simulink model "main_RI_LIEKF"  (R2023a)
settings: Solver=FixedStepAuto  StartTime=0.0  StopTime=220  FixedStep=0.01  RelTol=1e-3
InitFcn:
  | initNavigation0612_AOA;
values from neighbouring files (symbols this model uses):
  CF_enable = 0    [initNavigation.m]
  dt = 0.01    [initNavigation.m]
  dtDelay = -0.03    [initNavigation.m]
  g0 = 9.795    [initNavigation.m]
  gam0_rad = 0/57.3    (= 0)    [initNavigation.m]
  H_sensor_type = 0    [initNavigation.m]
  KF_enable = 1    [initNavigation.m]
  P0 = diag([1*ones(3,1);0.01*ones(3,1);0.1*ones(3,1);0.001*ones(3,1);0.00001*ones(3,1)])    [initNavigation.m]
  P0_RIEKF = diag([1*ones(3,1);0.01*ones(3,1);0.1*ones(3,1);0.001*ones(3,1);0.00001*ones(3,1);      0.01*ones(3,1);[0;2;2]/57.3;[0.1;0.1;0.1]])^2    [initNavigation.m]
  pd0 = 0    [initNavigation.m]
  pe0 = 0    [initNavigation.m]
  phi0_rad = 0/57.3    (= 0)    [initNavigation.m]
  pn0 = 0    [initNavigation.m]
  psi = -178    [initNavigation.m]
  psi0_rad = 0/57.3    (= 0)    [initNavigation.m]
  state_dim = 24    [initNavigation.m]
  Time = 0:0.01:(size(traindata.AttackAngle,1) - 1)*0.01    [NNLiftCoefficientFit.m]
  vd0 = 0    [initNavigation.m]
  ve0 = 0    [initNavigation.m]
  vn0 = 0    [initNavigation.m]
undefined symbols (not defined in the file or in its folder): DiscIntNeverNeededParam, Discrete, INS_CONST, INS_EXPORT, INS_PARAM, magnitude, p, param, pInitialization, sys
libraries: simulink x69, simulink_extras x64, dspstat3 x56, sharedtransform x49, ctrlSharedLib x36, sharedTrackingLibrary x17, FMT_Model_Lib x13, matrix_library x12, deeplib x4, dspsolvers x4, vrlib x4, aerolibconvert2 x1
(part 18 of 22)

== system main_RI_LIEKF/State estimation/distribute CF/distribute CF/Translation_estimate/V_Horizontal_estimation/Rxy_kalman filter1/Vxy kalman filter/kalman/Subsystem ==
  F : Inport
  G : Inport  Port=2
  Q : Inport  Port=3
  X : Inport  Port=4
  P : Inport  Port=5
  Add : Sum
  Math Function3 : Math  Operator=transpose  SignedPower=on
  Math Function4 : Math  Operator=transpose  SignedPower=on
  MatrixMultiply : Product  Multiplication=Matrix(*)
  MatrixMultiply1 : Product  Inputs=3  Multiplication=Matrix(*)
  MatrixMultiply8 : Product  Inputs=3  Multiplication=Matrix(*)
  Xk_k_1 : Outport
  Pk_k_1 : Outport  Port=2
  wires:
  [Pk_k_1] -> Pk_k_1/1
  [Xk_k_1] -> Xk_k_1/1
  P/1 -> [P]
  X/1 -> [X]
  Q/1 -> [Q]
  G/1 -> [G]
  F/1 -> [F]
  [F] -> MatrixMultiply/1
  [G] -> Math Function4/1
  [X] -> MatrixMultiply/2
  MatrixMultiply8/1 -> Add/2
  [G] -> MatrixMultiply8/1
  Add/1 -> [Pk_k_1]
  [F] -> MatrixMultiply1/1
  [P] -> MatrixMultiply1/2
  Math Function3/1 -> MatrixMultiply1/3
  [F] -> Math Function3/1
  MatrixMultiply1/1 -> Add/1
  MatrixMultiply/1 -> [Xk_k_1]
  [Q] -> MatrixMultiply8/2
  Math Function4/1 -> MatrixMultiply8/3

== system main_RI_LIEKF/State estimation/distribute CF/distribute CF/Translation_estimate/V_Horizontal_estimation/Rxy_kalman filter1/Vxy kalman filter/kalman/Subsystem1 ==
  note: 计算卡尔曼增益Kk
  Xkk : Inport
  Pkk : Inport  Port=2
  H : Inport  Port=3
  R : Inport  Port=4
  Z : Inport  Port=5
  Enable : EnablePort
  Add2 : Sum
  Add3 : Sum  Inputs=+-
  Add4 : Sum  Inputs=+-
  Add5 : Sum
  Constant : Constant  Value=eye(4)  OutDataTypeStr=single
  LDL Solver1 : dspsolvers/LDL Solver  errmode=Warning
      settings: RTWMemSecFuncInitTerm=Default  RTWMemSecFuncExecute=Default  RTWMemSecDataConstants=Default  RTWMemSecDataInternal=Default  RTWMemSecDataParameters=Default
  Math Function5 : Math  Operator=transpose  SignedPower=on
  Math Function6 : Math  Operator=transpose  SignedPower=on
  MatrixMultiply{4..7,9..10} (6 alike) : Product  Multiplication=Matrix(*)
  Scope : Scope
  POut : Outport
  XOut : Outport  Port=2
  wires:
  Pkk/1 -> [Pk_k_1]
  Z/1 -> [Z]
  Xkk/1 -> [Xk_k_1]
  Add2/1 -> XOut/1
  H/1 -> [H]
  MatrixMultiply6/1 -> Add4/2
  Add5/1 -> LDL Solver1/1
  R/1 -> [R]
  [Pk_k_1] -> MatrixMultiply7/2
  [Xk_k_1] -> MatrixMultiply9/2
  [H] -> MatrixMultiply9/1
  [H] -> MatrixMultiply6/2
  [Xk_k_1] -> Add2/1
  [Kk] -> MatrixMultiply6/1
  Constant/1 -> Add4/1
  [R] -> Add5/2
  [Pk_k_1] -> MatrixMultiply10/2
  [H] -> Math Function5/1
  LDL Solver1/1 -> Math Function6/1
  MatrixMultiply5/1 -> Add5/1
  MatrixMultiply10/1 -> LDL Solver1/2, MatrixMultiply5/1
  [Z] -> Add3/1
  [Kk] -> MatrixMultiply4/1
  MatrixMultiply4/1 -> Add2/2
  Add4/1 -> MatrixMultiply7/1
  Math Function6/1 -> [Kk], Scope/1
  Math Function5/1 -> MatrixMultiply5/2
  Add3/1 -> MatrixMultiply4/2
  [H] -> MatrixMultiply10/1
  MatrixMultiply7/1 -> POut/1
  MatrixMultiply9/1 -> Add3/2

== system main_RI_LIEKF/State estimation/distribute CF/distribute CF/AHRS1/Correct/Attitude_Correction/Attitude_Correct/Acc_Correct/Verticle_Correct/Saturation ==
  u : Inport
  Constant1 : Constant  Value=1e-4  OutDataTypeStr=Inherit: Inherit via back propagation
  Divide : Product  Inputs=**/
  Divide1 : Product  Inputs=*/
  Divide2 : Product  Inputs=**
  MinMax : MinMax  Function=max  Inputs=2
  Saturation : Saturate  UpperLimit=pi/2  LowerLimit=-pi/2
  Trigonometric Function : Trigonometry
  Vector Modulus : FMT_Model_Lib/Math/Vector Modulus
  max : Constant  Value=10/180*pi  OutDataTypeStr=single
  y : Outport
  wires:
  Constant1/1 -> MinMax/2
  Saturation/1 -> Trigonometric Function/1
  u/1 -> Vector Modulus/1, Divide/1
  Trigonometric Function/1 -> Divide2/1
  Divide/1 -> y/1
  Vector Modulus/1 -> Divide1/1, MinMax/1
  Divide1/1 -> Saturation/1
  Divide2/1 -> Divide/2
  max/1 -> Divide1/2, Divide2/2
  MinMax/1 -> Divide/3

== system main_RI_LIEKF/State estimation/distribute CF/distribute CF/AHRS1/Correct/Attitude_Correction/Attitude_Correct/Acc_Estimator/Measure_Acc/Bus_Selection ==
  Sensor_Data : Inport
  Bus Selector2 : BusSelector  OutputSignals=GPS_Data.vn_mPs,GPS_Data.ve_mPs,GPS_Data.vd_mPs
  Mux : Mux  Inputs=3
  gps_vel_O_mPs : Outport
  wires:
  Sensor_Data/1 -> Bus Selector2/1
  Bus Selector2/1 -> Mux/1  "<vn_mPs>"
  Bus Selector2/2 -> Mux/2  "<ve_mPs>"
  Bus Selector2/3 -> Mux/3  "<vd_mPs>"
  Mux/1 -> gps_vel_O_mPs/1

== system main_RI_LIEKF/State estimation/distribute CF/distribute CF/AHRS1/Correct/Attitude_Correction/Attitude_Correct/Acc_Estimator/Measure_Acc/GPS_Meas_Acc ==
  reset : Inport
  gps_vel_O_mPs : Inport  Port=2
  Enable : EnablePort  StatesWhenEnabling=reset
  Integrator : DiscreteIntegrator  ExternalReset=level  SampleTime=-1  ICPrevOutput=DiscIntNeverNeededParam  ICPrevScaledInput=DiscIntNeverNeededParam
  Integrator1 : DiscreteIntegrator  ExternalReset=level  InitialConditionSource=external  SampleTime=-1  ICPrevOutput=DiscIntNeverNeededParam  ICPrevScaledInput=DiscIntNeverNeededParam
  Sum : Sum  Inputs=|++
  Sum1 : Sum  Inputs=|+-
  gain : Gain  Gain=2*zeta*fc
  gain1 : Gain  Gain=fc^2
  gps_acc_O_mPs2 : Outport
  wires:
  Integrator1/1 -> Sum1/2
  Integrator/1 -> gps_acc_O_mPs2/1, Sum/2
  reset/1 -> Integrator1/2, Integrator/2
  gain/1 -> Sum/1
  Sum1/1 -> gain/1, gain1/1
  Sum/1 -> Integrator1/1
  gps_vel_O_mPs/1 -> Sum1/1, Integrator1/3
  gain1/1 -> Integrator/1

== system main_RI_LIEKF/State estimation/distribute CF/distribute CF/AHRS1/Correct/Attitude_Correction/Attitude_Correct/Acc_Estimator/Measure_Acc/Valid_Check ==
  Sensor_Data : Inport
  Bus Selector : BusSelector  OutputSignals=GPS_Data.GPS_valid,GPS_Data.spd_quality
  Logical Operator1 : Logic  AllPortsSameDT=off  OutDataTypeStr=boolean
  Relay : Relay  OnSwitchValue=0.2  OffSwitchValue=0.1
  gps_meas_acc_valid : Outport
  wires:
  Sensor_Data/1 -> Bus Selector/1
  Logical Operator1/1 -> gps_meas_acc_valid/1
  Bus Selector/1 -> Logical Operator1/1  "<GPS_valid>"
  Relay/1 -> Logical Operator1/2
  Bus Selector/2 -> Relay/1  "<spd_quality>"

== system main_RI_LIEKF/State estimation/distribute CF/distribute CF/Correct/Attitude_Correction/Attitude_Correct/Acc_Correct/Verticle_Correct/Saturation/norm ==
  In1 : Inport
  Sqrt : Sqrt
  Square : Math  Operator=square  SignedPower=on
  Sum of Elements : Sum  Inputs=+
  Out1 : Outport
  wires:
  Sum of Elements/1 -> Sqrt/1
  Square/1 -> Sum of Elements/1
  Sqrt/1 -> Out1/1
  In1/1 -> Square/1

== system main_RI_LIEKF/State estimation/distribute CF/distribute CF/Correct/Attitude_Correction/Attitude_Correct/Subsystem2/gps_meas_acc-加速度估计/TD_baro/Subsystem ==
  In1 : Inport
  Constant1 : Constant  Value=dt  OutDataTypeStr=single
  Constant3 : Constant  Value=0.23  OutDataTypeStr=single
  Constant4 : Constant  Value=900  OutDataTypeStr=single
  Delay1 : Delay  DelayLength=1  InitialConditionSource=Input port
      settings: InputPortMap=u0,p4
  MATLAB Function2 : MATLAB Function  TreatAsAtomicUnit=on
  Memory : Memory  InheritSampleTime=on
  Scope : Scope  NumInputPorts=3
  u2 : Outport
  wires:
  In1/1 -> MATLAB Function2/2(u0), Delay1/2, Scope/1
  Constant1/1 -> MATLAB Function2/1(T)
  MATLAB Function2/1(u1) -> Delay1/1
  Memory/1 -> Scope/2, MATLAB Function2/4("u2 ")
  Constant3/1 -> MATLAB Function2/5(h)
  Delay1/1 -> MATLAB Function2/3("u1 "), Scope/3
  MATLAB Function2/2(u2) -> u2/1, Memory/1
  Constant4/1 -> MATLAB Function2/6(r)

== system main_RI_LIEKF/State estimation/distribute CF/distribute CF/Correct/Attitude_Correction/Attitude_Correct/Subsystem2/gps_meas_acc-加速度估计/TD_baro/Subsystem1 ==
  In1 : Inport
  Constant1 : Constant  Value=dt  OutDataTypeStr=single
  Constant3 : Constant  Value=0.23  OutDataTypeStr=single
  Constant4 : Constant  Value=900  OutDataTypeStr=single
  Delay1 : Delay  DelayLength=1  InitialConditionSource=Input port
      settings: InputPortMap=u0,p4
  MATLAB Function2 : MATLAB Function  TreatAsAtomicUnit=on
  Memory : Memory  InheritSampleTime=on
  Scope : Scope  NumInputPorts=3
  u2 : Outport
  wires:
  Constant4/1 -> MATLAB Function2/6(r)
  MATLAB Function2/2(u2) -> u2/1, Memory/1
  Delay1/1 -> Scope/3, MATLAB Function2/3("u1 ")
  Constant3/1 -> MATLAB Function2/5(h)
  Memory/1 -> MATLAB Function2/4("u2 "), Scope/2
  MATLAB Function2/1(u1) -> Delay1/1
  Constant1/1 -> MATLAB Function2/1(T)
  In1/1 -> Scope/1, Delay1/2, MATLAB Function2/2(u0)

== system main_RI_LIEKF/State estimation/distribute CF/distribute CF/Correct/Attitude_Correction/Attitude_Correct/Subsystem2/gps_meas_acc-加速度估计/TD_baro/Subsystem2 ==
  In1 : Inport
  Constant1 : Constant  Value=dt  OutDataTypeStr=single
  Constant3 : Constant  Value=0.23  OutDataTypeStr=single
  Constant4 : Constant  Value=900  OutDataTypeStr=single
  Delay1 : Delay  DelayLength=1  InitialConditionSource=Input port
      settings: InputPortMap=u0,p4
  MATLAB Function2 : MATLAB Function  TreatAsAtomicUnit=on
  Memory : Memory  InheritSampleTime=on
  Scope : Scope  NumInputPorts=3
  u2 : Outport
  wires:
  In1/1 -> MATLAB Function2/2(u0), Delay1/2, Scope/1
  Constant1/1 -> MATLAB Function2/1(T)
  MATLAB Function2/1(u1) -> Delay1/1
  Memory/1 -> Scope/2, MATLAB Function2/4("u2 ")
  Constant3/1 -> MATLAB Function2/5(h)
  Delay1/1 -> MATLAB Function2/3("u1 "), Scope/3
  MATLAB Function2/2(u2) -> u2/1, Memory/1
  Constant4/1 -> MATLAB Function2/6(r)

== matlab function main_RI_LIEKF/State estimation/15dim KF1/Error State Kalman Filter/MATLAB Function2 ==
  data: P output
function P=P0
    g0 = 9.7803267714;       % 重力加速度
    %t=0.01;                  %采样时间
    sec = 4.848136811095360e-06;
    Re = 6378137;
    dph = 4.848136811095360e-06;
    ug = 9.780326771399999e-06;

    %角度随机游走系数(度/小时)
    % web=[3;3;3]*(pi/180)/3600;
     %web=[6;6;6]*sec;
     web= [2.908882086657216e-07;2.908882086657216e-07;2.908882086657216e-07];
    %速度随机游走系数（米/s/sqrt（小时））
     %wdb=[500;500;500]*ug;
    wdb=[9.780326771400000e-06;9.780326771400000e-06;9.780326771400000e-06];

    %sqg=[1;1;1]*(pi/180)/3600;
    %sqa=[1;1;1]*1e-6*g0;
    
    sqg=zeros(3,1);
    sqa=zeros(3,1);
    %系统噪声协方差矩阵
    %kf.Qt = diag([imuerr.web; imuerr.wdb; zeros(3,1); imuerr.sqg; imuerr.sqa; zeros(3,1)])^2;
 %Q=diag([web;wdb;zeros(3,1);sqg;sqa;w_GPS_V;w_GPS_R])^2;
%  Q=diag([web;wdb;zeros(3,1);sqg;sqa])^2;
  P = diag([1*ones(3,1);0.1*ones(3,1);[0.001;0.001;0.01];0.001*ones(3,1);0.1*ones(3,1)]);
%P = 1e-3^2*ones(15,1);
%Q = diag([8.461594994075240e-10*[1;1;1];9.565479175536352e-09*[1;1;1];zeros(15,1)]);
end

== matlab function main_RI_LIEKF/State estimation/15dim KF1/INS propogation/Init_PVQ2/Horizontal_attitude/Hem2JPL ==
  data: q input; y output
function y = fcn(q)

y = [q(2:4);q(1)];

== matlab function main_RI_LIEKF/State estimation/15dim KF1/INS propogation/Init_PVQ2/Horizontal_attitude/Hem2JPL1 ==
  data: q input; y output
function y = fcn(q)

y = [q(2:4);q(1)];

== matlab function main_RI_LIEKF/State estimation/15dim KF1/INS propogation/att_update/JPLQuatMult ==
  data: quatA input; q_t output; quatB input
function q_t = QuatMult(quatA,quatB)
% Calculate the following quaternion product quatA * quatB using the 
% standard identity 
%{
inline Eigen::Matrix<double, 4, 1> quat_multiply(const Eigen::Matrix<double, 4, 1> &q, const Eigen::Matrix<double, 4, 1> &p) {
  Eigen::Matrix<double, 4, 1> q_t;
  Eigen::Matrix<double, 4, 4> Qm;
  // create big L matrix
  Qm.block(0, 0, 3, 3) = q(3, 0) * Eigen::MatrixXd::Identity(3, 3) - skew_x(q.block(0, 0, 3, 1));
  Qm.block(0, 3, 3, 1) = q.block(0, 0, 3, 1);
  Qm.block(3, 0, 1, 3) = -q.block(0, 0, 3, 1).transpose();
  Qm(3, 3) = q(3, 0);
  q_t = Qm * p;
  // ensure unique by forcing q_4 to be >0
  if (q_t(3, 0) < 0) {
    q_t *= -1;
  }
  // normalize and return
  return q_t / q_t.norm();
}
%}
Qm = zeros(4,4);
q_t = zeros(4,1);
Qm(1:3,1:3) = quatA(4)*eye(3,3) - skewMat(quatA(1:3));
Qm(1:3,4) = quatA(1:3);
Qm(4,1:3) = -quatA(1:3)';
Qm(4,4) = quatA(4);
q_t = Qm * quatB;
if q_t(4) < 0
    q_t = q_t * (-1);
end
q_t = q_t / norm(q_t);
end

== matlab function main_RI_LIEKF/State estimation/15dim KF1/INS propogation/att_update/JPLQuatMult1 ==
  data: quatA input; q_t output; quatB input
function q_t = QuatMult(quatA,quatB)
% Calculate the following quaternion product quatA * quatB using the 
% standard identity 
%{
inline Eigen::Matrix<double, 4, 1> quat_multiply(const Eigen::Matrix<double, 4, 1> &q, const Eigen::Matrix<double, 4, 1> &p) {
  Eigen::Matrix<double, 4, 1> q_t;
  Eigen::Matrix<double, 4, 4> Qm;
  // create big L matrix
  Qm.block(0, 0, 3, 3) = q(3, 0) * Eigen::MatrixXd::Identity(3, 3) - skew_x(q.block(0, 0, 3, 1));
  Qm.block(0, 3, 3, 1) = q.block(0, 0, 3, 1);
  Qm.block(3, 0, 1, 3) = -q.block(0, 0, 3, 1).transpose();
  Qm(3, 3) = q(3, 0);
  q_t = Qm * p;
  // ensure unique by forcing q_4 to be >0
  if (q_t(3, 0) < 0) {
    q_t *= -1;
  }
  // normalize and return
  return q_t / q_t.norm();
}
%}
Qm = zeros(4,4);
q_t = zeros(4,1);
Qm(1:3,1:3) = quatA(4)*eye(3,3) - skewMat(quatA(1:3));
Qm(1:3,4) = quatA(1:3);
Qm(4,1:3) = -quatA(1:3)';
Qm(4,4) = quatA(4);
q_t = Qm * quatB;
if q_t(4) < 0
    q_t = q_t * (-1);
end
q_t = q_t / norm(q_t);
end

== matlab function main_RI_LIEKF/State estimation/15dim KF1/INS propogation/att_update/JPLrv2q ==
  data: rotVec input; quaternion output
% convert froma rotation vector in radians to a quaternion
function quaternion = RotToQuat(rotVec)

vecLength = sqrt(rotVec(1)^2 + rotVec(2)^2 + rotVec(3)^2);

if vecLength < 1e-6
  quaternion = [0;0;0;1];
else
  quaternion = [rotVec/vecLength*sin(0.5*vecLength);cos(0.5*vecLength);];
end

== matlab function main_RI_LIEKF/State estimation/15dim KF1/INS propogation/att_update/JPLrv2q1 ==
  data: deltaTheta input; updateQuat output
% convert froma rotation vector in radians to a quaternion
function updateQuat = RotToQuat(deltaTheta)

    deltaq = 0.5 * deltaTheta;
    
    checkNorm = deltaq' * deltaq;
    
    if checkNorm > 1
        updateQuat = [deltaq; 1];
        updateQuat = updateQuat / sqrt(1 + checkNorm);
    else
        updateQuat = [deltaq; sqrt(1 - checkNorm)];
    end
    
    updateQuat = updateQuat / norm(updateQuat);
end

== matlab function main_RI_LIEKF/State estimation/15dim KF1/INS propogation/att_update/MATLAB Function1 ==
  data: q input; Rot output
function Rot = quat_2_Rot(q)

%{
inline Eigen::Matrix<double, 3, 3> quat_2_Rot(const Eigen::Matrix<double, 4, 1> &q) {
  Eigen::Matrix<double, 3, 3> q_x = skew_x(q.block(0, 0, 3, 1));
  Eigen::MatrixXd Rot = (2 * std::pow(q(3, 0), 2) - 1) * Eigen::MatrixXd::Identity(3, 3) - 2 * q(3, 0) * q_x +
                        2 * q.block(0, 0, 3, 1) * (q.block(0, 0, 3, 1).transpose());
  return Rot;
}
%}
q_x = skewMat(q(1:3));
Rot = (2 * q(4)^2 - 1) * eye(3, 3) - 2 * q(4) * q_x +...
       2 * q(1:3) * q(1:3)';
end

== matlab function main_RI_LIEKF/State estimation/RI EKF/INS propogation/AOA//SA//Vwind update/Subsystem/LSTM predict1/MATLAB Function5 ==
  data: X input; X_nYPred output
function X_nYPred = LSTMnet(X)
    sig_X = [0.2380; 0.1523 ;0.0429;0.1379];
    sig_Y = 0.0690;
    mu_X = [0.0068;-0.0055;-0.0070;-0.0450];
    mu_Y = -0.0228;
    X_norm = (X - mu_X) ./ sig_X;
    persistent X_nYPredorm_store;
    if isempty(X_nYPredorm_store)
        X_nYPredorm_store = zeros(1000,4);
    end

    X_nYPredorm_store = [X_nYPredorm_store(2:end,:);X_norm'];
    %[~,YPred_seq] = predictAndUpdateState(net.net,X_nYPredorm_store);
     X_nYPred = single(X_nYPredorm_store);
    % YPred_seq = predict(net.net,X_nYPredorm_store');
    % YPred_test = YPred_seq(end);
    % YPred_test = double(YPred_test* sig_Y + mu_Y)*57.3;

end

== matlab function main_RI_LIEKF/State estimation/ER EKF/INS propogation/Init_PVQ/Horizontal_attitude/Hem2JPL ==
  data: q input; y output
function y = fcn(q)

y = [q(2:4);q(1)];

== matlab function main_RI_LIEKF/State estimation/ER EKF/INS propogation/Init_PVQ/Horizontal_attitude/Hem2JPL1 ==
  data: q input; y output
function y = fcn(q)

y = [q(2:4);q(1)];

== matlab function main_RI_LIEKF/State estimation/0609bk/Error State Kalman Filter/Extended Kalman Filter1/Output/MATLAB Function ==
  data: S input; P output
function P = fcn(S)
    
    % Get back Covariance from Square-root Covariance
    P = S*S';
    
end

== matlab function main_RI_LIEKF/State estimation/ER EKF/INS propogation/att_update/JPLQuatMult ==
  data: quatA input; q_t output; quatB input
function q_t = QuatMult(quatA,quatB)
% Calculate the following quaternion product quatA * quatB using the 
% standard identity 
%{
inline Eigen::Matrix<double, 4, 1> quat_multiply(const Eigen::Matrix<double, 4, 1> &q, const Eigen::Matrix<double, 4, 1> &p) {
  Eigen::Matrix<double, 4, 1> q_t;
  Eigen::Matrix<double, 4, 4> Qm;
  // create big L matrix
  Qm.block(0, 0, 3, 3) = q(3, 0) * Eigen::MatrixXd::Identity(3, 3) - skew_x(q.block(0, 0, 3, 1));
  Qm.block(0, 3, 3, 1) = q.block(0, 0, 3, 1);
  Qm.block(3, 0, 1, 3) = -q.block(0, 0, 3, 1).transpose();
  Qm(3, 3) = q(3, 0);
  q_t = Qm * p;
  // ensure unique by forcing q_4 to be >0
  if (q_t(3, 0) < 0) {
    q_t *= -1;
  }
  // normalize and return
  return q_t / q_t.norm();
}
%}
Qm = zeros(4,4);
q_t = zeros(4,1);
Qm(1:3,1:3) = quatA(4)*eye(3,3) - skewMat(quatA(1:3));
Qm(1:3,4) = quatA(1:3);
Qm(4,1:3) = -quatA(1:3)';
Qm(4,4) = quatA(4);
q_t = Qm * quatB;
if q_t(4) < 0
    q_t = q_t * (-1);
end
q_t = q_t / norm(q_t);
end

== matlab function main_RI_LIEKF/State estimation/ER EKF/INS propogation/att_update/JPLQuatMult1 ==
  data: quatA input; q_t output; quatB input
function q_t = QuatMult(quatA,quatB)
% Calculate the following quaternion product quatA * quatB using the 
% standard identity 
%{
inline Eigen::Matrix<double, 4, 1> quat_multiply(const Eigen::Matrix<double, 4, 1> &q, const Eigen::Matrix<double, 4, 1> &p) {
  Eigen::Matrix<double, 4, 1> q_t;
  Eigen::Matrix<double, 4, 4> Qm;
  // create big L matrix
  Qm.block(0, 0, 3, 3) = q(3, 0) * Eigen::MatrixXd::Identity(3, 3) - skew_x(q.block(0, 0, 3, 1));
  Qm.block(0, 3, 3, 1) = q.block(0, 0, 3, 1);
  Qm.block(3, 0, 1, 3) = -q.block(0, 0, 3, 1).transpose();
  Qm(3, 3) = q(3, 0);
  q_t = Qm * p;
  // ensure unique by forcing q_4 to be >0
  if (q_t(3, 0) < 0) {
    q_t *= -1;
  }
  // normalize and return
  return q_t / q_t.norm();
}
%}
Qm = zeros(4,4);
q_t = zeros(4,1);
Qm(1:3,1:3) = quatA(4)*eye(3,3) - skewMat(quatA(1:3));
Qm(1:3,4) = quatA(1:3);
Qm(4,1:3) = -quatA(1:3)';
Qm(4,4) = quatA(4);
q_t = Qm * quatB;
if q_t(4) < 0
    q_t = q_t * (-1);
end
q_t = q_t / norm(q_t);
end

== matlab function main_RI_LIEKF/State estimation/ER EKF/INS propogation/att_update/JPLrv2q ==
  data: rotVec input; quaternion output
% convert froma rotation vector in radians to a quaternion
function quaternion = RotToQuat(rotVec)

vecLength = sqrt(rotVec(1)^2 + rotVec(2)^2 + rotVec(3)^2);

if vecLength < 1e-6
  quaternion = [0;0;0;1];
else
  quaternion = [rotVec/vecLength*sin(0.5*vecLength);cos(0.5*vecLength);];
end

== matlab function main_RI_LIEKF/State estimation/ER EKF/INS propogation/att_update/JPLrv2q1 ==
  data: deltaTheta input; updateQuat output
% convert froma rotation vector in radians to a quaternion
function updateQuat = RotToQuat(deltaTheta)

    deltaq = 0.5 * deltaTheta;
    
    checkNorm = deltaq' * deltaq;
    
    if checkNorm > 1
        updateQuat = [deltaq; 1];
        updateQuat = updateQuat / sqrt(1 + checkNorm);
    else
        updateQuat = [deltaq; sqrt(1 - checkNorm)];
    end
    
    updateQuat = updateQuat / norm(updateQuat);
end

== matlab function main_RI_LIEKF/State estimation/ER EKF/INS propogation/att_update/MATLAB Function1 ==
  data: q input; Rot output
function Rot = quat_2_Rot(q)

%{
inline Eigen::Matrix<double, 3, 3> quat_2_Rot(const Eigen::Matrix<double, 4, 1> &q) {
  Eigen::Matrix<double, 3, 3> q_x = skew_x(q.block(0, 0, 3, 1));
  Eigen::MatrixXd Rot = (2 * std::pow(q(3, 0), 2) - 1) * Eigen::MatrixXd::Identity(3, 3) - 2 * q(3, 0) * q_x +
                        2 * q.block(0, 0, 3, 1) * (q.block(0, 0, 3, 1).transpose());
  return Rot;
}
%}
q_x = skewMat(q(1:3));
Rot = (2 * q(4)^2 - 1) * eye(3, 3) - 2 * q(4) * q_x +...
       2 * q(1:3) * q(1:3)';
end

== matlab function main_RI_LIEKF/State estimation/bak1/Error State Kalman Filter/Simulink Function - State Transition Jacobian/Cal Phi/MATLAB Function1 ==
  data: axyz input; Phi output; Cnb input; wxyz input; dt input
function Phi = fcn(axyz, Cnb, wxyz,dt)
    
    %{
    F.block(0, 0, 3, 3) = exp_so3(-w_hat * dt);
        F.block(0, 9, 3, 3).noalias() = -exp_so3(-w_hat * dt) * Jr_so3(-w_hat * dt) * dt;
        F.block(9, 9, 3, 3).setIdentity();
        F.block(6, 0, 3, 3).noalias() = -R_Gtoi.transpose() * skew_x(a_hat * dt);
        F.block(6, 6, 3, 3).setIdentity();
        F.block(6, 12, 3, 3) = -R_Gtoi.transpose() * dt;
        F.block(12, 12, 3, 3).setIdentity();
        F.block(3, 0, 3, 3).noalias() = -0.5 * R_Gtoi.transpose() * skew_x(a_hat * dt * dt);
        F.block(3, 6, 3, 3) = Eigen::Matrix3d::Identity() * dt;
        F.block(3, 12, 3, 3) = -0.5 * R_Gtoi.transpose() * dt * dt;
        F.block(3, 3, 3, 3).setIdentity();
        Eigen::Matrix<double, 15, 12> G = Eigen::Matrix<double, 15, 12>::Zero();
    %}
    Phi = zeros(18,18);
    % 
    Phi(1:3,1:3) = eye(3);      %P-P
    Phi(1:3,4:6) = dt * eye(3); %P-V
    Phi(1:3,7:9) = -0.5*Cnb'*skewMat(axyz * dt * dt); %P-the
    % 
    Phi(4:6,4:6) = eye(3);
    Phi(4:6,7:9) = -Cnb' * skewMat(axyz * dt);
    Phi(4:6,10:12) = -Cnb'*dt ;
    % 
    Phi(7:9,7:9) = exp_so3(-wxyz * dt);     %the-the
    Phi(7:9,13:15) = -exp_so3(-wxyz * dt) * Jl_so3(wxyz * dt) * dt; %the-bias g
    % 
    Phi(10:12,10:12) = eye(3);
    % % 
    Phi(13:15,13:15) = eye(3);
    % 
    Phi(1:3,10:12) = - 0.5*Cnb' * dt * dt;
    Phi(16:18,16:18) = eye(3);
end

== matlab function main_RI_LIEKF/State estimation/bak1/Error State Kalman Filter/Simulink Function - State Transition Jacobian/MATLAB Function ==
  data: Cnb input; G output; wxyz input; dt input
function G = fcn(Cnb, wxyz, dt)
    % G.block(0, 0, 3, 3) = -exp_so3(-w_hat * dt) * Jr_so3(-w_hat * dt) * dt;
    %    G.block(6, 3, 3, 3) = -R_Gtoi.transpose() * dt;
    %    G.block(3, 3, 3, 3) = -0.5 * R_Gtoi.transpose() * dt * dt;
    %    G.block(9, 6, 3, 3).setIdentity();
    %    G.block(12, 9, 3, 3).setIdentity();
    
    G = zeros(18,15);
    G(7:9,4:6) = -exp_so3(-wxyz * dt) * Jl_so3(wxyz * dt) * dt;
    G(1:3,1:3) = -0.5 * Cnb' * dt * dt;
    G(4:6,1:3) = -Cnb' * dt;
    G(10:12,7:9) = eye(3);
    G(13:15,10:12) = eye(3);
    G(13:15,10:12) = eye(3);
    G(16:18,13:15) = eye(3);
    G(16:18,1:3) = -eye(3);
end

== matlab function main_RI_LIEKF/State estimation/bak1/INS propogation/att_update/MATLAB Function ==
  data: Rbn_k_1 input; Rbn output; w input; dt input
function Rbn = fcn(Rbn_k_1, w, dt)
    Rbn = Rbn_k_1 * exp_so3(w * dt);
end

== matlab function main_RI_LIEKF/State estimation/bak1/INS propogation/att_update/MATLAB Function2 ==
  data: delta input; Rbn_correct output single size=[3,3]; Rbn input
function Rbn_correct = fcn(delta, Rbn)
    Rbn_correct = zeros(3,3);
    Rbn_correct = exp_so3(delta)* Rbn;
end

== matlab function main_RI_LIEKF/Sensor_Data_Process/IMU_Data_Process/accl_preprocessing2/MATLAB Function1 ==
  data: curr_input input; curr_output output single; sample_freq input; cutoff_freq input
function curr_output = second_LPF_Butter_x(curr_input,sample_freq,cutoff_freq)
   persistent input_x;
   persistent output_x;

   if isempty(input_x)
       input_x = [0;0;0];
   end
   
   if isempty(output_x)
       output_x = [0;0;0];
   end
    B = [0,0,0];
    A = [0,0,0];
    M_PI_F = 3.1415926;
	fr = sample_freq / cutoff_freq;
	ohm = tan( M_PI_F / fr );
	c = 1.0 + 2.0 * cos( M_PI_F / 4.0 ) * ohm + ohm * ohm;
	B(1) = ohm * ohm / c;
	B(2) = 2.0 * B(1);
	B(3) = B(1);
	A(1) = 2.0 * ( ohm * ohm - 1.0) / c;
	A(2) = (1.0 - 2.0 * cos( M_PI_F / 4.0 ) * ohm + ohm * ohm) / c;
	%/*获取最新输入*/
	input_x(3) = curr_input;
	%/* Butterworth */
	output_x(3) =B(1) * input_x(3) + B(2) * input_x(2) +B(3) * input_x(1) - A(1) * output_x(2) - A(2) * output_x(1);
	curr_output = single(output_x(3));
   % /* 输入序列保存 */
	input_x(1) = input_x(2);
	input_x(2) = input_x(3);
	%/*输出序列保存 */
	output_x(1) = output_x(2);
	output_x(2) = output_x(3);

== matlab function main_RI_LIEKF/State estimation/bak1/INS propogation/vel_pos_update/pos update/MATLAB Function ==
  data: dtheta input; pos_correct output single; KFState_dp input; pos input
function pos_correct = fcn(dtheta, KFState_dp, pos)
    
    pos_correct =  KFState_dp + exp_so3(dtheta)*pos;
end

== matlab function main_RI_LIEKF/State estimation/bak1/INS propogation/vel_pos_update/vel update/MATLAB Function ==
  data: dtheta input; vel_correct output single; KFState_dv input; vel input
function vel_correct = fcn(dtheta, KFState_dv, vel)
    
    vel_correct =  KFState_dv + exp_so3( dtheta)*vel;
end

== matlab function main_RI_LIEKF/State estimation/RI EKF/Error State Kalman Filter/bak/Simulink Function - State Transition Jacobian/Cal Phi1/MATLAB Function1 ==
  data: vn input; Phi output; pn input; Rbn input; dt input
function Phi = fcn(vn,pn, Rbn,dt)
    
    %{
    F.block(0, 0, 3, 3) = exp_so3(-w_hat * dt);
        F.block(0, 9, 3, 3).noalias() = -exp_so3(-w_hat * dt) * Jr_so3(-w_hat * dt) * dt;
        F.block(9, 9, 3, 3).setIdentity();
        F.block(6, 0, 3, 3).noalias() = -R_Gtoi.transpose() * skew_x(a_hat * dt);
        F.block(6, 6, 3, 3).setIdentity();
        F.block(6, 12, 3, 3) = -R_Gtoi.transpose() * dt;
        F.block(12, 12, 3, 3).setIdentity();
        F.block(3, 0, 3, 3).noalias() = -0.5 * R_Gtoi.transpose() * skew_x(a_hat * dt * dt);
        F.block(3, 6, 3, 3) = Eigen::Matrix3d::Identity() * dt;
        F.block(3, 12, 3, 3) = -0.5 * R_Gtoi.transpose() * dt * dt;
        F.block(3, 3, 3, 3).setIdentity();
        Eigen::Matrix<double, 15, 12> G = Eigen::Matrix<double, 15, 12>::Zero();
    %}
    %
    %
    %F = [0_33         0_33  0_33   -Rbn          0_33]
    %    [skew(gn)     0_33  0_33  -skew(vn)Rbn   -Rbn]
    %    [0.5*skew(gn) I_33  0_33  -skew(pn)Rbn   -Rbn]
    %    [         0_69                  I66          ]
    Phi = zeros(15,15);
    g0 = 9.79;
    gn = [0;0;-g0];
    F  = zeros(15,15);
    F(1:3,10:12) = -Rbn;
    F(4:6,1:3)   = skewMat(gn);
    F(4:6,10:12) = -skewMat(vn)*Rbn;
    F(4:6,13:15) = -Rbn;
    F(7:9,4:6)   = eye(3);
    F(7:9,1:3)   = 0.5*skewMat(gn) * dt;
    F(7:9,10:12) = -skewMat(pn)*Rbn;
    F(7:9,13:15) = -Rbn;
    %F(10:15,10:15) = eye(6);
    Phi = eye(15) + F * dt;

end

== matlab function main_RI_LIEKF/State estimation/RI EKF/Error State Kalman Filter/bak/Simulink Function - State Transition Jacobian/MATLAB Function1 ==
  data: Rbn input; G output; vn input; pn input; dt input
function G = fcn(Rbn, vn,pn, dt)
    % G.block(0, 0, 3, 3) = -exp_so3(-w_hat * dt) * Jr_so3(-w_hat * dt) * dt;
    %    G.block(6, 3, 3, 3) = -R_Gtoi.transpose() * dt;
    %    G.block(3, 3, 3, 3) = -0.5 * R_Gtoi.transpose() * dt * dt;
    %    G.block(9, 6, 3, 3).setIdentity();
    %    G.block(12, 9, 3, 3).setIdentity();

    G = zeros(15,12);
    % G(1:3,1:3) = -  Rbn * dt;
    % G(4:6,1:3) = -skewMat(vn)*Rbn* dt;
    % G(4:6,4:6) =  - Rbn;
    % G(7:9,1:3) = -skewMat(pn)*Rbn * dt;
    % G(7:9,4:6) =  - Rbn;
    % G(10:12,7:9) = eye(3)*dt;
    % G(13:15,10:12) = eye(3)*dt;
    G(1:3,1:3) =  - Rbn * dt;
    G(4:6,1:3) = -skewMat(vn)*Rbn * dt;
    G(4:6,4:6) =  - Rbn* dt;
    G(7:9,1:3) = -skewMat(pn)*Rbn * dt;
    G(7:9,4:6) =  - Rbn* dt;
    G(10:12,7:9) = eye(3) ;
    G(13:15,10:12) = eye(3) ;
    
    %G = G*double(dt);
end

== matlab function main_RI_LIEKF/State estimation/RI EKF/Error State Kalman Filter/Simulink Function - GPS Measurements1/MATLAB Function ==
  data: vn input; H_baro output; pn input
function H_baro = fcn(vn, pn)
    state_dim = 24;
    H = zeros(6,state_dim);
    H(1:3,1:3) = skewMat(vn);
    H(4:6,1:3) = skewMat(pn);
    H(1:6,4:9) = eye(6);
    
    A = [0 0 0 0 0 1];
    H_baro = A * H;
end

== matlab function main_RI_LIEKF/State estimation/RI EKF/Error State Kalman Filter/Simulink Function - GPS Measurements2/MATLAB Function ==
  data: Rbn input; Magn input; H output; dtheta input
function H = fcn(Rbn, Magn, dtheta)
    state_dim = 24;
    H = zeros(3,state_dim);
    H(1:3,1:3) =  Rbn * skewMat(Magn);
    H(1:3,16:18) =  Rbn * skewMat(dtheta);
end

== matlab function main_RI_LIEKF/State estimation/RI EKF/Error State Kalman Filter/Simulink Function - GPS Measurements3/MATLAB Function ==
  data: Rbn input; Rab input; H output; vn input; v_wind input
function H = fcn(Rbn,Rab, vn,v_wind)
    state_dim = 24;
    A = Rab' * Rbn';
    H = zeros(3,state_dim);
   % H(1:3,1:3) =  - skewMat(vn - v_wind);
   % H(1:3,4:6) =  eye(3);
    H(1:3,19:21) =  - skewMat(vn - v_wind);
    H(1:3,22:24) =  - eye(3);
    H = double(A * H);
end

== matlab function main_RI_LIEKF/State estimation/RI EKF/INS propogation/AOA//SA//Vwind update/Subsystem/MATLAB Function ==
  data: u input; Rab output
function Rab = fcn(u)
    Rab = zeros(3,3);
        ca = cos(u(2));
        sa = sin(u(2));
        cb = cos(u(3));
        sb = sin(u(3));
    Rab = double([ca * cb,-ca * sb, -sa;
        sb, cb, 0;
        sa * cb, -sa * sb, ca;]);
end

== matlab function main_RI_LIEKF/State estimation/RI EKF/INS propogation/AOA//SA//Vwind update/Subsystem/MATLAB Function2 ==
  data: delta input; Rbn_correct output double size=[3,3]; Rbn input
function Rbn_correct = fcn(delta, Rbn)
    delta(1) = 0;
    Rbn_correct = zeros(3,3);
     %Rbn_correct = exp_so3(delta)* Rbn;
    Rbn_correct =double(( eye(3) + skewMat(delta))* Rbn);
end

== matlab function main_RI_LIEKF/Sensor_Data_Process/Subsystem/TD_baro/MATLAB Function2 ==
  data: T input single; u1 output; u0 input; u1 input single; u2 input single; h input single; r input single; u2 output
function [u1,u2]=diff_TD_2(T,u0,u1,u2,h,r)
    %init
    %T是信号周期，u0原始信号输入，u1跟踪原始信号，u2原始信号差分值，
    %h滤波因子（h=T时接近一阶差分）越大滤波好延迟大；r速度因子，越大跟踪的越快但是噪声放大；

	x1=0; x2=0;
	delta=0;
	delta0=0;
	y=0;
	fabs_y=0;
	a0=0;
	a=0;
    fst=0;
    
	x1 = u1;
	x2 = u2;
	delta = r*h;
	delta0 = delta*h;
	y = x1 - u0 + h*x2;
	fabs_y = abs(y);   
	a0 = sqrt(delta*delta + 8 * r*fabs_y);
    
	if (fabs_y <= delta0)
		a = x2 + y / h;
    else
        a = x2 + 0.5*(a0 - delta)*sign(y);
    end
    
	if (abs(a) <= delta)
		fst = -r*a / delta;
    else
		fst = -r*sign(a);
    end
	u1 = single(x1 + T*x2); %计算跟踪信号
	u2 = single(x2 + T*fst); % 计算微分信号

== matlab function main_RI_LIEKF/State estimation/0609bk/Error State Kalman Filter/Extended Kalman Filter1/Predict/Predict ==
  settings: updateMethod=DISCRETE  sampleTime=SampleTime
  data: x input; xNew output; P input; Q input; uState input; unused input; P output; pS parameter
function [xNew,P] = fcn(x,P,Q,uState,~,pS)
% ekfCorrect Prediction step for EKF
%
%   Copyright 2016-2021 The MathWorks, Inc.

%#codegen

% If process noise is time-varying then compute square-root
% factorization.
if pS.HasTimeVaryingQ
   Q = matlabshared.tracking.internal.svdPSD(Q);
end

% Construct fcn handles
if pS.IsSimulinkFcn
    StateTransitionJacobianFcnH_SL = str2func(pS.FcnName);
    if pS.HasAdditiveNoise
        StateTransitionFcnH = @(fState)StateTransitionJacobianFcnH_SL(fState);
    else
        StateTransitionFcnH = @(fState,fProcNoise)StateTransitionJacobianFcnH_SL(fState,fProcNoise);
    end
else
    StateTransitionFcnH = str2func(pS.FcnName);
end
if pS.HasJacobian
    if pS.IsSimulinkFcn
        StateTransitionJacobianFcnH_SL = str2func(pS.JacobianFcnName);
        if pS.HasAdditiveNoise
            StateTransitionJacobianFcnH = @(fState)StateTransitionJacobianFcnH_SL(fState);
        else
            StateTransitionJacobianFcnH = @(fState,fProcNoise)StateTransitionJacobianFcnH_SL(fState,fProcNoise);
        end
    else
        StateTransitionJacobianFcnH = str2func(pS.JacobianFcnName);
    end
else
    StateTransitionJacobianFcnH = [];
end

switch pS.NumberOfExtraArgumentInports
    case 0
        extraArgs = {};
    case 1
        extraArgs = {uState};
    otherwise
        assert(false);
end

% Check if dimensions and type of State and Jacobian are correct
if pS.HasAdditiveNoise
   % Additive noise
   
   % StateTransitionFcn
   xTry = StateTransitionFcnH(x, extraArgs{:});
   
   if pS.IsSimulinkFcn
      hasError = any(size(x) ~= size(xTry));
   else
      hasError = any(size(x) ~= size(xTry)) || ~isa(xTry, class(x));
   end
   
   coder.internal.errorIf(...
      hasError,...
      'shared_tracking:ExtendedKalmanFilter:StateNonMatchingSizeOrClass',...
      'StateTransitionFcn', 'State', numel(x));
   
   if pS.HasJacobian
      % Jacobian
      F = StateTransitionJacobianFcnH(x, extraArgs{:});
      % F needs to be square
      isSizeNotCorrect = ~all(size(F) == numel(x));
      
      if pS.IsSimulinkFcn
         hasError = isSizeNotCorrect;
      else
         hasError = isSizeNotCorrect || ~isa(F, class(x));
      end
      
      coder.internal.errorIf(...
         hasError,...
         'shared_tracking:ExtendedKalmanFilter:StateTransitionJacobianNonMatchingSizeOrClass',...
         'StateTransitionJacobianFcn', numel(x));
   end
else
   % Non-additive noise
   
   % StateTransitionFcn
   xTry = StateTransitionFcnH(x, zeros(size(Q,1),1,'like',x),extraArgs{:});
   
   if pS.IsSimulinkFcn
      hasError = any(size(x) ~= size(xTry));
   else
      hasError = any(size(x) ~= size(xTry)) || ~isa(xTry, class(x));
   end
   
   coder.internal.errorIf(...
      hasError,...
      'shared_tracking:ExtendedKalmanFilter:StateNonMatchingSizeOrClass',...
      'StateTransitionFcn', 'State', numel(x))
   
   if pS.HasJacobian
      % Jacobian
      F = StateTransitionJacobianFcnH(x, zeros(size(Q,1),1,'like',x),extraArgs{:});
      % F needs to be square
      isSizeNotCorrect = ~all(size(F) == numel(x));
      
      if pS.IsSimulinkFcn
         hasError = isSizeNotCorrect;
      else
         hasError = isSizeNotCorrect || ~isa(F, class(x));
      end
       
      coder.internal.errorIf(...
         hasError,...
         'shared_tracking:ExtendedKalmanFilter:StateTransitionJacobianNonMatchingSizeOrClass',...
         'StateTransitionJacobianFcn', numel(x));
   end
end

xNew = zeros(size(x),'like',x); %#ok<PREALL>

if pS.HasAdditiveNoise
    [xNew,P] = matlabshared.tracking.internal.EKFPredictorAdditive.predict(...
        Q,x,P,StateTransitionFcnH,StateTransitionJacobianFcnH,extraArgs{:});
else    
    [xNew,P] = matlabshared.tracking.internal.EKFPredictorNonAdditive.predict(...
        Q,x,P,StateTransitionFcnH,StateTransitionJacobianFcnH,extraArgs{:});
end
end

== matlab function main_RI_LIEKF/State estimation/RI EKF/INS propogation/AOA//SA//Vwind update/Subsystem/LSTM predict1/MATLAB Function6 ==
  data: YPred_test input; YPred_test_out output
function YPred_test_out = LSTMnet(YPred_test)
    sig_X = [0.2380; 0.1523 ;0.0429;0.1379];
    sig_Y = 0.0690;
    mu_X = [0.0068;-0.0055;-0.0070;-0.0450];
    mu_Y = -0.0228;
    YPred_test_out = YPred_test(end);
    YPred_test_out = single(YPred_test_out* sig_Y + mu_Y)*57.3;

end

== matlab function main_RI_LIEKF/State estimation/LI EKF1/Error State Kalman Filter/Cal Q1/MATLAB Function1 ==
  data: Q output; dt input
function Q = fcn(dt)
    % G.block(0, 0, 3, 3) = -exp_so3(-w_hat * dt) * Jr_so3(-w_hat * dt) * dt;
    %    G.block(6, 3, 3, 3) = -R_Gtoi.transpose() * dt;
    %    G.block(3, 3, 3, 3) = -0.5 * R_Gtoi.transpose() * dt * dt;
    %    G.block(9, 6, 3, 3).setIdentity();
    %    G.block(12, 9, 3, 3).setIdentity();
    

    cov_dim = 21;
    Q = zeros(cov_dim,cov_dim);
%     noises_sigma_a_2 = 2.0000e-4^2;
%     noises_sigma_w_2 = 1.6968e-4^2;
%     noises_sigma_ab_2 = 3.0000e-4^2;
%     noises_sigma_wb_2 = 1.9393e-5^2;
    noises_sigma_a_2 = 0.001^2*1;
    %noises_sigma_w_2 = 0.0001^2;
    noises_sigma_w_2 = 0.0001^2;
    noises_sigma_ab_2 = 1.0000e-4^2*1;
    noises_sigma_wb_2 = 0.00002^2;
    noises_sigma_mb_2 = 0.001^2;
    noises_sigma_dtheta_2 = (1/57.3)^2;
    noises_sigma_dwind_2 = 0.01^2;
    Q = diag([noises_sigma_w_2 / dt * ones(3,1); ...
                noises_sigma_a_2 / dt * ones(3,1); ...
                noises_sigma_wb_2 * dt * ones(3,1); ...
                noises_sigma_ab_2 * dt * ones(3,1); ...
                noises_sigma_mb_2 * dt * ones(3,1); ...
                noises_sigma_dtheta_2 * ones(3,1); ...
                noises_sigma_dwind_2* ones(3,1)]);
    

end

== matlab function main_RI_LIEKF/State estimation/LI EKF1/Error State Kalman Filter/Extended Kalman Filter1/Correct1/Correct ==
  settings: updateMethod=DISCRETE  sampleTime=SampleTime
  data: x input; xNew output; P input; P output; yMeas input; R input; uMeas input; blockOrdering input; pM parameter; blockOrdering output
function [xNew,P,blockOrdering] = fcn(x,P,yMeas,R,uMeas,blockOrdering,pM)
% ekfCorrect Correction step for EKF
%
%   Copyright 2016-2021 The MathWorks, Inc.

%#codegen

% If measurement noise is time-varying then compute square-root
% factorization.
if pM.HasTimeVaryingR
   R = matlabshared.tracking.internal.svdPSD(R);
end

% Construct the function handle for measurement fcn
if pM.IsSimulinkFcn
    MeasurementFcnH_SL = str2func(pM.FcnName);
    if pM.HasAdditiveNoise
        MeasurementFcnH = @(fState)MeasurementFcnH_SL(fState);
    else
        MeasurementFcnH = @(fState,fMeasNoise)MeasurementFcnH_SL(fState,fMeasNoise);
    end
else
    MeasurementFcnH = str2func(pM.FcnName);
end

% Construct the function handle for measurement Jacobian fcn
if pM.HasJacobian
    if pM.IsSimulinkFcn
        MeasurementJacobianFcnH_SL = str2func(pM.JacobianFcnName);
        if pM.HasAdditiveNoise
            MeasurementJacobianFcnH = @(fState)MeasurementJacobianFcnH_SL(fState);
        else
            MeasurementJacobianFcnH = @(fState,fMeasNoise)MeasurementJacobianFcnH_SL(fState,fMeasNoise);
        end
    else
        MeasurementJacobianFcnH = str2func(pM.JacobianFcnName);
    end
else
    MeasurementJacobianFcnH = [];
end

% Handle (optional) extra input arguments of the measurement & jacobian fcns
switch pM.NumberOfExtraArgumentInports
    case 0
        extraArgs = {};
    case 1
        extraArgs = {uMeas};
    otherwise
        assert(false);
end

% Construct the corrector, perform the update
if pM.HasAdditiveNoise
    ekfCorrector = matlabshared.tracking.internal.EKFCorrectorAdditive();
else
    ekfCorrector = matlabshared.tracking.internal.EKFCorrectorNonAdditive();
end

% Check if dimensions and type of Measurement and Jacobian are correct
if pM.HasAdditiveNoise
   % Additive noise
   
   % MeasurementFcn
   ztry = MeasurementFcnH(x, extraArgs{:});
   
   if pM.IsSimulinkFcn
      hasError = (numel(ztry) ~= numel(yMeas));
   else
      hasError = (numel(ztry) ~= numel(yMeas)) || ~isa(ztry, class(x));
   end
   
   coder.internal.errorIf(...
      hasError,...
      'shared_tracking:ExtendedKalmanFilter:MeasurementNonMatchingSizeOrClass',...
      'MeasurementFcn');
   
   if pM.HasJacobian
      % MeasurementJacobianFcn
      Htry = MeasurementJacobianFcnH(x, extraArgs{:});
      isSizeNotCorrect = numel(yMeas) ~= size(Htry,1) || numel(x) ~= size(Htry,2);
      
      if pM.IsSimulinkFcn
         hasError = isSizeNotCorrect;
      else
         hasError = isSizeNotCorrect || ~isa(Htry, class(x));
      end
      
      coder.internal.errorIf(...
         hasError,...
         'shared_tracking:ExtendedKalmanFilter:MeasurementJacobianNonMatchingSizeOrClass',...
         'MeasurementJacobianFcn',numel(yMeas),numel(x));
   end   
else
   % Non-additive noise
   
   % MeasurementFcn
   ztry = MeasurementFcnH(...
      x, zeros(size(R,1),1,'like',x), ...
      extraArgs{:});   

   if pM.IsSimulinkFcn
      hasError = (numel(ztry) ~= numel(yMeas));
   else
      hasError = (numel(ztry) ~= numel(yMeas)) || ~isa(ztry, class(x));
   end
   
   coder.internal.errorIf(...
      hasError,...
      'shared_tracking:ExtendedKalmanFilter:MeasurementNonMatchingSizeOrClass',...
      'MeasurementFcn');
   
   if pM.HasJacobian
      % MeasurementJacobianFcn
      Htry = MeasurementJacobianFcnH(...
         x, zeros(size(R,1),1,'like',x), ...
         extraArgs{:});
      
      isSizeNotCorrect = numel(yMeas) ~= size(Htry,1) || numel(x) ~= size(Htry,2);     
      
      if pM.IsSimulinkFcn
         hasError = isSizeNotCorrect;
      else
         hasError = isSizeNotCorrect || ~isa(Htry, class(x));
      end
      
      coder.internal.errorIf(...
         hasError,...
         'shared_tracking:ExtendedKalmanFilter:MeasurementJacobianNonMatchingSizeOrClass',...
         'MeasurementJacobianFcn',numel(yMeas),numel(x));
   end
end
% Measurement wrapping
ekfCorrector.HasMeasurementWrapping = pM.HasWrapping;

xNew = zeros(size(x),'like',x); %#ok<PREALL>
% wk = 0;
[xNew,P] = ekfCorrector.correct(...
        yMeas,R,x,P,MeasurementFcnH,MeasurementJacobianFcnH,extraArgs{:});
end

== matlab function main_RI_LIEKF/State estimation/LI EKF1/Error State Kalman Filter/Extended Kalman Filter1/Correct1/IGG_check/MATLAB Function ==
  data: err input; w output; k0 input; k1 input; zk0 input; zk1 input
function w = fcn(err,k0,k1,zk0,zk1)
    err = abs(err);  w = err;
    for k=1:2
        if err(k)<=k0,    w(k)=1;
        elseif err(k)>k1, w(k)=0;
        else,             w(k)=k0/err(k);  
        end
    end
        if err(3)<=zk0,    w(3)=1;
        elseif err(3)>zk1, w(3)=0;
        else,             w(3)=zk0/err(3);  
        end
end

== matlab function main_RI_LIEKF/State estimation/LI EKF1/Error State Kalman Filter/Extended Kalman Filter1/Output/MATLAB Function ==
  data: S input; P output
function P = fcn(S)
    
    % Get back Covariance from Square-root Covariance
    P = S*S';
    
end

== matlab function main_RI_LIEKF/State estimation/LI EKF1/Error State Kalman Filter/Extended Kalman Filter1/Predict/Predict ==
  settings: updateMethod=DISCRETE  sampleTime=SampleTime
  data: x input; xNew output; P input; Q input; uState input; unused input; P output; pS parameter
function [xNew,P] = fcn(x,P,Q,uState,~,pS)
% ekfCorrect Prediction step for EKF
%
%   Copyright 2016-2021 The MathWorks, Inc.

%#codegen

% If process noise is time-varying then compute square-root
% factorization.
if pS.HasTimeVaryingQ
   Q = matlabshared.tracking.internal.svdPSD(Q);
end

% Construct fcn handles
if pS.IsSimulinkFcn
    StateTransitionJacobianFcnH_SL = str2func(pS.FcnName);
    if pS.HasAdditiveNoise
        StateTransitionFcnH = @(fState)StateTransitionJacobianFcnH_SL(fState);
    else
        StateTransitionFcnH = @(fState,fProcNoise)StateTransitionJacobianFcnH_SL(fState,fProcNoise);
    end
else
    StateTransitionFcnH = str2func(pS.FcnName);
end
if pS.HasJacobian
    if pS.IsSimulinkFcn
        StateTransitionJacobianFcnH_SL = str2func(pS.JacobianFcnName);
        if pS.HasAdditiveNoise
            StateTransitionJacobianFcnH = @(fState)StateTransitionJacobianFcnH_SL(fState);
        else
            StateTransitionJacobianFcnH = @(fState,fProcNoise)StateTransitionJacobianFcnH_SL(fState,fProcNoise);
        end
    else
        StateTransitionJacobianFcnH = str2func(pS.JacobianFcnName);
    end
else
    StateTransitionJacobianFcnH = [];
end

switch pS.NumberOfExtraArgumentInports
    case 0
        extraArgs = {};
    case 1
        extraArgs = {uState};
    otherwise
        assert(false);
end

% Check if dimensions and type of State and Jacobian are correct
if pS.HasAdditiveNoise
   % Additive noise
   
   % StateTransitionFcn
   xTry = StateTransitionFcnH(x, extraArgs{:});
   
   if pS.IsSimulinkFcn
      hasError = any(size(x) ~= size(xTry));
   else
      hasError = any(size(x) ~= size(xTry)) || ~isa(xTry, class(x));
   end
   
   coder.internal.errorIf(...
      hasError,...
      'shared_tracking:ExtendedKalmanFilter:StateNonMatchingSizeOrClass',...
      'StateTransitionFcn', 'State', numel(x));
   
   if pS.HasJacobian
      % Jacobian
      F = StateTransitionJacobianFcnH(x, extraArgs{:});
      % F needs to be square
      isSizeNotCorrect = ~all(size(F) == numel(x));
      
      if pS.IsSimulinkFcn
         hasError = isSizeNotCorrect;
      else
         hasError = isSizeNotCorrect || ~isa(F, class(x));
      end
      
      coder.internal.errorIf(...
         hasError,...
         'shared_tracking:ExtendedKalmanFilter:StateTransitionJacobianNonMatchingSizeOrClass',...
         'StateTransitionJacobianFcn', numel(x));
   end
else
   % Non-additive noise
   
   % StateTransitionFcn
   xTry = StateTransitionFcnH(x, zeros(size(Q,1),1,'like',x),extraArgs{:});
   
   if pS.IsSimulinkFcn
      hasError = any(size(x) ~= size(xTry));
   else
      hasError = any(size(x) ~= size(xTry)) || ~isa(xTry, class(x));
   end
   
   coder.internal.errorIf(...
      hasError,...
      'shared_tracking:ExtendedKalmanFilter:StateNonMatchingSizeOrClass',...
      'StateTransitionFcn', 'State', numel(x))
   
   if pS.HasJacobian
      % Jacobian
      F = StateTransitionJacobianFcnH(x, zeros(size(Q,1),1,'like',x),extraArgs{:});
      % F needs to be square
      isSizeNotCorrect = ~all(size(F) == numel(x));
      
      if pS.IsSimulinkFcn
         hasError = isSizeNotCorrect;
      else
         hasError = isSizeNotCorrect || ~isa(F, class(x));
      end
       
      coder.internal.errorIf(...
         hasError,...
         'shared_tracking:ExtendedKalmanFilter:StateTransitionJacobianNonMatchingSizeOrClass',...
         'StateTransitionJacobianFcn', numel(x));
   end
end

xNew = zeros(size(x),'like',x); %#ok<PREALL>

if pS.HasAdditiveNoise
    [xNew,P] = matlabshared.tracking.internal.EKFPredictorAdditive.predict(...
        Q,x,P,StateTransitionFcnH,StateTransitionJacobianFcnH,extraArgs{:});
else    
    [xNew,P] = matlabshared.tracking.internal.EKFPredictorNonAdditive.predict(...
        Q,x,P,StateTransitionFcnH,StateTransitionJacobianFcnH,extraArgs{:});
end
end

== matlab function main_RI_LIEKF/State estimation/LI EKF1/Error State Kalman Filter/MATLAB Function ==
  data: u input; dp output size=3; dv output size=3; dtheta output size=3; da output size=3; dg output size=3; dm output size=3; dtheta_a output size=3; dv_wind output size=3
function [dp,dv,dtheta,da,dg,dm,dtheta_a,dv_wind] = fcn(u)
    dtheta = u(1:3);
    dv = u(4:6);
    dp = u(7:9);
    dg = u(10:12);
    da = u(13:15);
    dm = u(16:18);
    dtheta_a = u(19:21);
    dv_wind = u(22:24);
end

== matlab function main_RI_LIEKF/State estimation/LI EKF1/Error State Kalman Filter/Simulink Function - GPS Measurements/MATLAB Function ==
  data: vn input; H output; pn input
function H = fcn(vn, pn)
    state_dim = 24;
    H = zeros(6,state_dim);
    % H(1:3,1:3) = skewMat(vn);
    % H(4:6,1:3) = skewMat(pn);
    H(1:6,4:9) = eye(6);
    %H = -H;
end

== matlab function main_RI_LIEKF/State estimation/LI EKF1/Error State Kalman Filter/Simulink Function - GPS Measurements/MATLAB Function1 ==
  data: Rbn input; vn input; X_inv output; pn input
function X_inv = invX(Rbn, vn, pn)
    X_inv = zeros(5,5);
    Rnb = Rbn';
    X_inv(1:3,1:3) = Rnb;
    X_inv(1:3,4) = -Rnb * vn;
    X_inv(1:3,5) = -Rnb * pn;
    X_inv(4:5,4:5) = eye(2);
end

== matlab function main_RI_LIEKF/State estimation/RI EKF/Error State Kalman Filter/Cal Q1/MATLAB Function1 ==
  data: Q output; dt input
function Q = fcn(dt)
    % G.block(0, 0, 3, 3) = -exp_so3(-w_hat * dt) * Jr_so3(-w_hat * dt) * dt;
    %    G.block(6, 3, 3, 3) = -R_Gtoi.transpose() * dt;
    %    G.block(3, 3, 3, 3) = -0.5 * R_Gtoi.transpose() * dt * dt;
    %    G.block(9, 6, 3, 3).setIdentity();
    %    G.block(12, 9, 3, 3).setIdentity();
    

    cov_dim = 21;
    Q = zeros(cov_dim,cov_dim);
%     noises_sigma_a_2 = 2.0000e-4^2;
%     noises_sigma_w_2 = 1.6968e-4^2;
%     noises_sigma_ab_2 = 3.0000e-4^2;
%     noises_sigma_wb_2 = 1.9393e-5^2;
    noises_sigma_a_2 = 0.001^2*1;
    %noises_sigma_w_2 = 0.0001^2;
    noises_sigma_w_2 = 0.0001^2;
    noises_sigma_ab_2 = 1.0000e-4^2*1;
    noises_sigma_wb_2 = 0.00002^2;
    noises_sigma_mb_2 = 0.001^2;
    noises_sigma_dtheta_2 = (1/57.3)^2;
    noises_sigma_dwind_2 = 0.01^2;
    Q = diag([noises_sigma_w_2 / dt * ones(3,1); ...
                noises_sigma_a_2 / dt * ones(3,1); ...
                noises_sigma_wb_2 * dt * ones(3,1); ...
                noises_sigma_ab_2 * dt * ones(3,1); ...
                noises_sigma_mb_2 * dt * ones(3,1); ...
                noises_sigma_dtheta_2 * ones(3,1); ...
                noises_sigma_dwind_2* ones(3,1)]);
end
